simulink model "ATV_LAB4_SIMU_Q5"  (R2017b)
settings: Solver=VariableStepAuto  StartTime=0.0  StopTime=100  RelTol=1e-3
settings Model: Creator=Aluno  LastModifiedBy=Aluno

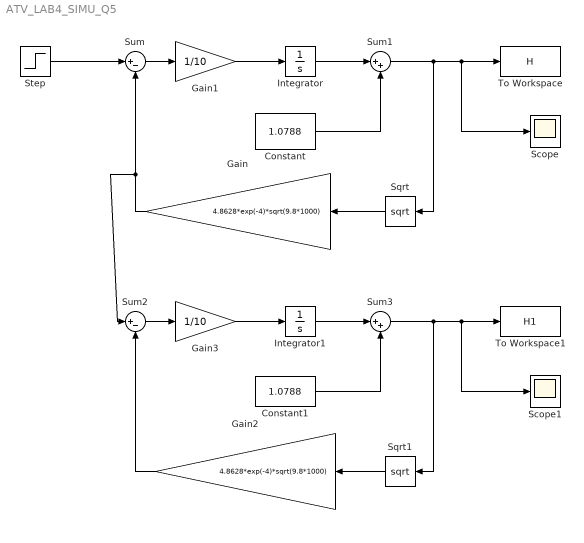
== system ATV_LAB4_SIMU_Q5 ==
  Constant : Constant  Value=1.0788
  Constant1 : Constant  Value=1.0788
  Gain : Gain  Gain=4.8628*exp(-4)*sqrt(9.8*1000)
  Gain1 : Gain  Gain=1/10
  Gain2 : Gain  Gain=4.8628*exp(-4)*sqrt(9.8*1000)
  Gain3 : Gain  Gain=1/10
  Integrator : Integrator
  Integrator1 : Integrator
  Scope : Scope
  Scope1 : Scope
  Sqrt : Sqrt  SaturateOnIntegerOverflow=on
  Sqrt1 : Sqrt  SaturateOnIntegerOverflow=on
  Step : Step  Time=0.04  Before=0.05  After=0.06  SampleTime=0
  Sum : Sum  Inputs=|+-
  Sum1 : Sum  Inputs=|++
  Sum2 : Sum  Inputs=|+-
  Sum3 : Sum  Inputs=|++
  To Workspace : ToWorkspace  VariableName=H  SampleTime=-1
  To Workspace1 : ToWorkspace  VariableName=H1  SampleTime=-1
  wires:
  Sum1/1 -> Sqrt/1, Scope/1, To Workspace/1
  Step/1 -> Sum/1
  Constant/1 -> Sum1/2
  Integrator/1 -> Sum1/1
  Gain1/1 -> Integrator/1
  Sum/1 -> Gain1/1
  Sqrt/1 -> Gain/1
  Gain/1 -> Sum2/1, Sum/2
  Gain2/1 -> Sum2/2
  Sqrt1/1 -> Gain2/1
  Sum2/1 -> Gain3/1
  Gain3/1 -> Integrator1/1
  Integrator1/1 -> Sum3/1
  Constant1/1 -> Sum3/2
  Sum3/1 -> To Workspace1/1, Scope1/1, Sqrt1/1
